simulink model "Simulation"  (R2022b)
settings: Solver=FixedStepAuto  StartTime=0.0  StopTime=param.Tsim  FixedStep=param.tSample  RelTol=1e-3
StopFcn:
  | run animation
  | run plotSol
undefined symbols (not defined in the file or in its folder): f, filterFr, filterFw, filterMr, FR_neg, FR_pos, g1, g2, g3, kFr, ki, kiSeil, kMr, kp, kpSeil, kVSl, kVSx, MR, MRP, param, xi_0
libraries: simulink x10, spsFirstOrderFilterLib x2
(part 3 of 3)

== matlab function Simulation/Flatness-based control1/feedforward control/MATLAB Function ==
  data: z1 input; u1 output; dz1 input; ddz1 input; d3z1 input; z2 input; dz2 input; ddz2 input; d3z2 input; u2 output
function [u1, u2] = feedforward_control(z1, dz1, ddz1, d3z1, z2, dz2, ddz2, d3z2)
%#codegen
% Inputs:
% z1, dz1, ddz1, d3z1: 
% z2, dz2, ddz2, d3z2: 
% Output:
% u1, u2: 


g = 9.81; 


l = z2 / sqrt(1 - (dz1 / dz2)^2); 


dl = (dz2 * sqrt(1 - (dz1 / dz2)^2) - (z2 * dz1 / dz2^2) * (-dz1 * ddz2 + dz2 * ddz1) / sqrt(1 - (dz1 / dz2)^2)) / (1 - (dz1 / dz2)^2);


ddl_num = ...
    ddz2 * sqrt(1 - (dz1 / dz2)^2) ...
    - dz2 * (dz1 / dz2^2) * (-dz1 * ddz2 + dz2 * ddz1) / sqrt(1 - (dz1 / dz2)^2) ...
    - z2 * ((-ddz1 * dz2 + dz1 * ddz2) / dz2^2)^2 ...
    + z2 * (-dz1 / dz2^2) * (-d3z1 * dz2 + 2 * ddz1 * ddz2 - dz1 * d3z2) / sqrt(1 - (dz1 / dz2)^2);
ddl = ddl_num / (1 - (dz1 / dz2)^2);


u1 = d3z1; 


u2 = (1 / l) * ( ...
      -g * (dz1 / dz2) ...  
      - ddz2 * sqrt(1 - (dz1 / dz2)^2) ... 
      - 2 * dz2^2 * dl ...
      - d3z2 * l ... 
      - ddl); 
end

== matlab function Simulation/Flatness-based control1/quasistatic tracking control/Computation of the flat output/MATLAB Function ==
  data: x1 input; z1 output; z2 output; x3 input; x5 input
function [z1, z2] = z(x1, x3, x5)
    % Compute flat outputs
    z1 = x1 + x3 * sin(x5);
    z2 = x3 * cos(x5);
end

== matlab function Simulation/Flatness-based control/trajectory generators/desired trajectory: SP change ==
  data: t input; z1_soll output; T input; z10 input; z20 input; z1T input; z2T input; z2_soll output
function [z1_soll, z2_soll] = fcn(t, T, z10, z20, z1T, z2T)
% Generate smooth trajectory for a single setpoint change
%
% Eingangsvariablen:
% t:    Current simulation time
% T:    Total duration of the trajectory
% z10:  Initial horizontal position
% z20:  Initial vertical position
% z1T:  Target horizontal position
% z2T:  Target vertical position
%
% Ausgangsvariablen:
% z1_soll:  Horizontal trajectory [z1, dz1, ddz1, ...]
% z2_soll:  Vertical trajectory [z2, dz2, ddz2, ...]

% Initialize output variables
z1_soll = zeros(1, 4); % [Position, Velocity, Acceleration, Jerk]
z2_soll = zeros(1, 4);

% Normalize time
tau = t / T; % Scaled time (0 <= tau <= 1)

% Ensure tau is within [0, 1] (handle cases where t > T)
if tau > 1
    tau = 1;
end

% Polynomial coefficients for a fifth-order polynomial
P = [6, -15, 10, 0, 0, 0]; % Standard polynomial for smooth interpolation

% Compute z1 trajectory and its derivatives
z1_soll(1) = z10 + (z1T - z10) * polyval(P, tau); % Position
z1_soll(2) = (z1T - z10) * polyval(polyder(P), tau) / T; % Velocity
z1_soll(3) = (z1T - z10) * polyval(polyder(polyder(P)), tau) / T^2; % Acceleration
z1_soll(4) = (z1T - z10) * polyval(polyder(polyder(polyder(P))), tau) / T^3; % Jerk

% Compute z2 trajectory and its derivatives
z2_soll(1) = z20 + (z2T - z20) * polyval(P, tau); % Position
z2_soll(2) = (z2T - z20) * polyval(polyder(P), tau) / T; % Velocity
z2_soll(3) = (z2T - z20) * polyval(polyder(polyder(P)), tau) / T^2; % Acceleration
z2_soll(4) = (z2T - z20) * polyval(polyder(polyder(polyder(P))), tau) / T^3; % Jerk
end

== matlab function Simulation/Flatness-based control1/quasistatic tracking control/Computation of the flat output/MATLAB Function1 ==
  data: dz1 output; dz2 output; x2 input; x3 input; x4 input; x5 input; x6 input
function [dz1, dz2] = dz(x2, x3, x4, x5, x6)
    dz1 = x2 + x4 * sin(x5) + x3 * x6 * cos(x5);
    dz2 = x4 * cos(x5) - x3 * x6 * sin(x5);
end

== matlab function Simulation/Flatness-based control1/quasistatic tracking control/Computation of the flat output/MATLAB Function2 ==
  data: x3 input; x5 input; x6 input; ddz1 output; ddz2 output; u1 input; u2 input
function [ddz1, ddz2] = ddz(x3, x5, x6, u1, u2)
g=9.81;
    ddz1 = sin(x5) * (u2 + u1 * sin(x5) - x3 * x6^2) - g * sin(x5) * cos(x5);
    ddz2 = cos(x5) * (u2 + u1 * sin(x5) - x3 * x6^2) + g * sin(x5)^2;
end

== matlab function Simulation/System model/Referenzmodell/Unterlagerte v-Regelung/Unterlagerte Regelung Seil/Gravitationskompensation ==
  data: m input; Mg output; g input; rho input
function Mg = fcn(m, g, rho)

Mg = m*g*rho;

== matlab function Simulation/Plot/Lastposition ==
  data: xW input; xL output; l input; phi input; yL output
function [xL, yL] = fcn(xW, l, phi)
    
    xL = xW + sin(phi)*l;
    yL = cos(phi)*l;

end

== matlab function Simulation/Flatness-based control1/quasistatic tracking control/Tracking controller/MATLAB Function ==
  data: ddz1 input; dddz1 input; v1 input; z2 input; u1 output; dz2 input; v2 input; dv2 input; u2 output; ddv2 input
function [u1, u2] = controlInputs(ddz1, dddz1, v1, z2, dz2, v2, dv2, ddv2)
    g = 9.81;
    
    A = (dz2*ddz1 + z2*dddz1)*(v2 - g);
    dA = (v2*ddz1 + dz2*dddz1*2 + z2*v1) * (v2 - g) + (dz2*ddz1 + z2*dddz1) * dv2;
    B = (A - z2*ddz1*dv2) / ((v2 - g)^2);
    dB = ((dA - dz2*ddz1*dv2 - z2*dddz1*dv2 - z2*ddz1*ddv2) * ((v2 - g)^2) ...
        - (A - z2*ddz1*dv2) * 2*(v2 - g)*dv2) ...
        / ((v2 - g)^4);
    x3 = sqrt(z2^2 + (z2*ddz1/(v2 - g))^2);
    dx3 = (2*z2*dz2 + B) / x3;

    u1 = ddz1 - dB;
    u2 = ((2*dz2*dz2 + 2*z2*v2 + dB)*x3...
        - (2*z2*dz2 + B)*dx3)...
        / (x3^2);
end

== matlab function Simulation/Flatness-based control1/quasistatic tracking control/Tracking controller/Tracking controller v1 for xLoad/MATLAB Function ==
  data: z1_star input; dz1_star input; ddz1_star input; dddz1_star input; d4z1_star input; z1 input; v1 output; dz1 input; ddz1 input; dddz1 input; pX01 input; pX02 input; pX03 input; pX04 input
function v1 = newInput_v1(z1_star, dz1_star, ddz1_star, dddz1_star, d4z1_star, z1, dz1, ddz1, dddz1, pX01, pX02, pX03, pX04)
    v1 = d4z1_star - pX01 * (dddz1 - dddz1_star) - pX02 * (ddz1 - ddz1_star) - pX03 * (dz1 - dz1_star) - pX04 * (z1 - z1_star);
end

== matlab function Simulation/Flatness-based control1/quasistatic tracking control/Tracking controller/Tracking controller v2 for yLoad/MATLAB Function ==
  data: z2_star input; dz2_star input; ddz2_star input; dddz2_star input; d4z2_star input; z2 input; v2 output; dz2 input; pY01_QS input; pY02_QS input; dv2 output; ddv2 output
function [v2, dv2, ddv2] = newInput_v2(z2_star, dz2_star, ddz2_star, dddz2_star, d4z2_star, z2, dz2, pY01_QS, pY02_QS)
    v2 = ddz2_star - pY01_QS * (dz2 - dz2_star) - pY02_QS * (z2 - z2_star);
    dv2 = dddz2_star - pY01_QS * (v2 - ddz2_star) - pY02_QS * (dz2 - dz2_star);
    ddv2 = d4z2_star - pY01_QS * (dv2 - dddz2_star) - pY02_QS * (v2 - ddz2_star);
end

== matlab function Simulation/Flatness-based control1/trajectory generators/desired trajectory: Parabola ==
  data: t input; z1_soll output; T input; z10 input; z1T input; a2 input; a1 input; z2_soll output; a0 input
function [z1_soll, z2_soll] = fcn(t, T, z10, z1T, a2, a1, a0)
% Parabola trajectory generator for avoiding obstacles
%
% Eingangsvariablen:
% t:        Current time
% T:        Duration of the trajectory
% z10:      Initial x-coordinate (horizontal position)
% z1T:      Final x-coordinate (horizontal position)
% a2, a1, a0: Coefficients of the parabolic equation z2 = a2*z1^2 + a1*z1 + a0
%
% Ausgangsvariablen:
% z1_soll:  Horizontal trajectory [z1, dz1, ddz1, ...]
% z2_soll:  Vertical trajectory [z2, dz2, ddz2, ...]

% Initialize output variables
z1_soll = zeros(1, 4); % [Position, Velocity, Acceleration, Jerk]
z2_soll = zeros(1, 4);

% Normalize time
tau = t / T; % Scaled time (0 <= tau <= 1)

% Boundary conditions for z1 (horizontal trajectory)
z1_start = z10;
z1_end = z1T;

% Polynomial coefficients for a fifth-order polynomial for z1
P_z1 = [6, -15, 10, 0, 0, 0]; % Scaled polynomial for smooth interpolation

% Compute z1 trajectory and its derivatives
z1_soll(1) = z1_start + (z1_end - z1_start) * polyval(P_z1, tau);
z1_soll(2) = (z1_end - z1_start) * polyval(polyder(P_z1), tau) / T;
z1_soll(3) = (z1_end - z1_start) * polyval(polyder(polyder(P_z1)), tau) / T^2;
z1_soll(4) = (z1_end - z1_start) * polyval(polyder(polyder(polyder(P_z1))), tau) / T^3;

% Compute z2 (vertical trajectory) based on the parabolic equation
z2_soll(1) = a2 * z1_soll(1)^2 + a1 * z1_soll(1) + a0; % Position
z2_soll(2) = 2 * a2 * z1_soll(1) * z1_soll(2) + a1 * z1_soll(2); % Velocity
z2_soll(3) = 2 * a2 * (z1_soll(2)^2 + z1_soll(1) * z1_soll(3)) + a1 * z1_soll(3); % Acceleration
z2_soll(4) = 2 * a2 * (2 * z1_soll(2) * z1_soll(3) + z1_soll(1) * z1_soll(4)) + a1 * z1_soll(4); % Jerk
end

== matlab function Simulation/Flatness-based control1/trajectory generators/desired trajectory: SP change ==
  data: t input; z1_soll output; T input; z10 input; z20 input; z1T input; z2T input; z2_soll output
function [z1_soll, z2_soll] = fcn(t, T, z10, z20, z1T, z2T)
% Generate smooth trajectory for a single setpoint change
%
% Eingangsvariablen:
% t:    Current simulation time
% T:    Total duration of the trajectory
% z10:  Initial horizontal position
% z20:  Initial vertical position
% z1T:  Target horizontal position
% z2T:  Target vertical position
%
% Ausgangsvariablen:
% z1_soll:  Horizontal trajectory [z1, dz1, ddz1, ...]
% z2_soll:  Vertical trajectory [z2, dz2, ddz2, ...]

% Initialize output variables
z1_soll = zeros(1, 4); % [Position, Velocity, Acceleration, Jerk]
z2_soll = zeros(1, 4);

% Normalize time
tau = t / T; % Scaled time (0 <= tau <= 1)

% Ensure tau is within [0, 1] (handle cases where t > T)
if tau > 1
    tau = 1;
end

% Polynomial coefficients for a fifth-order polynomial
P = [6, -15, 10, 0, 0, 0]; % Standard polynomial for smooth interpolation

% Compute z1 trajectory and its derivatives
z1_soll(1) = z10 + (z1T - z10) * polyval(P, tau); 
z1_soll(2) = (z1T - z10) * polyval(polyder(P), tau) / T; 
z1_soll(3) = (z1T - z10) * polyval(polyder(polyder(P)), tau) / T^2; 
z1_soll(4) = (z1T - z10) * polyval(polyder(polyder(polyder(P))), tau) / T^3; 

% Compute z2 trajectory and its derivatives
z2_soll(1) = z20 + (z2T - z20) * polyval(P, tau); 
z2_soll(2) = (z2T - z20) * polyval(polyder(P), tau) / T; 
z2_soll(3) = (z2T - z20) * polyval(polyder(polyder(P)), tau) / T^2; 
z2_soll(4) = (z2T - z20) * polyval(polyder(polyder(polyder(P))), tau) / T^3; 
end

== matlab function Simulation/Flatness-based control1/trajectory generators/desired trajectory: Sequence of SP changes ==
  data: t input; z1_soll output; T input; z10 input; z20 input; z2_soll output; T_task input; x_links input; x_rechts input; y_oben input; y_unten input
function [z1_soll, z2_soll] = fcn(t, T, z10, z20, T_task, x_links, x_rechts, y_oben, y_unten)
% Solltrajektoriengenerator für eine Folge von Arbeitspunktwechseln
%
%%%%%%%%%%%%%%%%%%%%%%%%%%%%%%%%%%%%%%%%%%%%%%%%%%%%%%%%%%%%%%%%%%%%%%%%%%%%%%%%%%%%%%%%%%%%%%
% Eingangsvariablen: 
% t:                    Zeit
% T:                    Zeitdauer eines Arbeitspunktwechsels
% T_task:               Zeitdauer zwischen dem Beginn zweier aufeinanderfolgender Arbeitspunktwechsel
% z10/z20:              Startsollzustand
% x_links, x_rechts:    x-Koordinate der linken/rechten Punkte
% y_oben, y_unten:      y-Koordinate der oberen/unteren Punkte
%
% Ausgangsvariablen:
% z1_soll:  Vektor [z1_soll, dz1_soll, ddz1_soll, ...]
% z2_soll:  Vektor [z2_soll, dz2_soll, ddz2_soll, ...]
%%%%%%%%%%%%%%%%%%%%%%%%%%%%%%%%%%%%%%%%%%%%%%%%%%%%%%%%%%%%%%%%%%%%%%%%%%%%%%%%%%%%%%%%%%%%%%

z1_soll = zeros(1, 4); 
z2_soll = zeros(1, 4);


setpoints = [
    z10, z20;              
    x_links, y_oben;       
    x_links, y_unten;       
    x_rechts, y_oben;       
    x_rechts, y_unten;     
    x_links, y_oben;       
    z10, z20                
];


n_segments = size(setpoints, 1) - 1;
segment_duration = T + T_task;


current_segment = floor(t / segment_duration) + 1;

if current_segment > n_segments
    z1_soll(1) = setpoints(end, 1);
    z2_soll(1) = setpoints(end, 2);
    return;
end

t_local = mod(t, segment_duration);


if t_local > T
    z1_soll(1) = setpoints(current_segment, 1);
    z2_soll(1) = setpoints(current_segment, 2);
    return;
end


z1_start = setpoints(current_segment, 1);
z2_start = setpoints(current_segment, 2);
z1_end = setpoints(current_segment + 1, 1);
z2_end = setpoints(current_segment + 1, 2);

tau = t_local / T;

P = [0, 0, 0, 35, -84, 70, 0, 0, 0, 0];


z1_soll(1) = z1_start + (z1_end - z1_start) * polyval(P, tau);
z1_soll(2) = (z1_end - z1_start) * polyval(polyder(P), tau) / T;
z1_soll(3) = (z1_end - z1_start) * polyval(polyder(polyder(P)), tau) / T^2;
z1_soll(4) = (z1_end - z1_start) * polyval(polyder(polyder(polyder(P))), tau) / T^3;


z2_soll(1) = z2_start + (z2_end - z2_start) * polyval(P, tau);
z2_soll(2) = (z2_end - z2_start) * polyval(polyder(P), tau) / T;
z2_soll(3) = (z2_end - z2_start) * polyval(polyder(polyder(P)), tau) / T^2;
z2_soll(4) = (z2_end - z2_start) * polyval(polyder(polyder(polyder(P))), tau) / T^3;
end

== matlab function Simulation/Flatness-based control/feedforward control/MATLAB Function ==
  data: z1 input; u1 output; dz1 input; ddz1 input; d3z1 input; z2 input; dz2 input; ddz2 input; d3z2 input; u2 output
function [u1, u2] = feedforward_control(z1, dz1, ddz1, d3z1, z2, dz2, ddz2, d3z2)
%#codegen
% Inputs:
% z1, dz1, ddz1, d3z1: 
% z2, dz2, ddz2, d3z2: 
% Output:
% u1, u2: 


g = 9.81; 


l = z2 / sqrt(1 - (dz1 / dz2)^2); 


dl = (dz2 * sqrt(1 - (dz1 / dz2)^2) - (z2 * dz1 / dz2^2) * (-dz1 * ddz2 + dz2 * ddz1) / sqrt(1 - (dz1 / dz2)^2)) / (1 - (dz1 / dz2)^2);


ddl_num = ...
    ddz2 * sqrt(1 - (dz1 / dz2)^2) ...
    - dz2 * (dz1 / dz2^2) * (-dz1 * ddz2 + dz2 * ddz1) / sqrt(1 - (dz1 / dz2)^2) ...
    - z2 * ((-ddz1 * dz2 + dz1 * ddz2) / dz2^2)^2 ...
    + z2 * (-dz1 / dz2^2) * (-d3z1 * dz2 + 2 * ddz1 * ddz2 - dz1 * d3z2) / sqrt(1 - (dz1 / dz2)^2);
ddl = ddl_num / (1 - (dz1 / dz2)^2);


u1 = d3z1; 


u2 = (1 / l) * ( ...
      -g * (dz1 / dz2) ...  
      - ddz2 * sqrt(1 - (dz1 / dz2)^2) ... 
      - 2 * dz2^2 * dl ...
      - d3z2 * l ... 
      - ddl); 
end

== matlab function Simulation/Plot1/Lastposition ==
  data: xW input; xL output; l input; phi input; yL output
function [xL, yL] = fcn(xW, l, phi)
    
    xL = xW + sin(phi)*l;
    yL = cos(phi)*l;

end

== matlab function Simulation/Plot1/yL_Beschraenkung (Parabel) ==
  data: xL input; yL_const output; p0 input; p1 input; p2 input
function yL_const  = fcn(xL, p0, p1, p2)
    % Quadratisches Polynom für die Zustandsbeschränkung p2*x^2+p1*x+p0 (im Horner Schema)
    yL_const = xL * ( p1 + (p2 * xL)) + p0;

end

== matlab function Simulation/System model1/Kinematisches Modell/sys_dgl  ==
  data: x input; u input; dx output
function dx = fcn(x,u)

dx = zeros(length(x), 1);
g = 9.81;

dx(1) = x(2);
dx(2) = u(1);
dx(3) = x(4);
dx(4) = u(2);
dx(5) = x(6);
dx(6) = -((g * sin(x(5)) + cos(x(5))*u(1) + 2 * x(4) * x(6)) / x(3));

== matlab function Simulation/System model1/Referenzmodell/Unterlagerte v-Regelung/Unterlagerte Regelung Seil/Gravitationskompensation ==
  data: m input; Mg output; g input; rho input
function Mg = fcn(m, g, rho)

Mg = m*g*rho;

== matlab function Simulation/System model1/Referenzmodell/Unterlagerte v-Regelung/Unterlagerte Regelung Seil/MATLAB Function7 ==
  data: muT input; c_TT input; c_HT input; omega_0 input; ldt input; Rho input; Mr output
function Mr = fcn(muT, c_TT, c_HT, omega_0, ldt, Rho)


Mr = -(muT*(-ldt/Rho)+c_TT*sign(-ldt/Rho)+(c_HT-c_TT)*sign(-ldt/Rho)*exp((-ldt^2*omega_0^2)/Rho^2));

% Mr = -(muT*(-ldt/Rho));

== matlab function Simulation/System model1/Referenzmodell/Unterlagerte v-Regelung/Unterlagerte Regelung Wagen/MATLAB Function2 ==
  data: mu_W_pos input; c_TW_pos input; c_HW_pos input; v_0_pos input; xdt input; Fr output
function Fr = fcn(mu_W_pos, c_TW_pos, c_HW_pos, v_0_pos, xdt)

%     Fr = -(mu_W_pos*xdt +(c_HW_pos-c_TW_pos)*sign(xdt)*exp(-xdt^2/v_0_pos^2) + c_TW_pos*sign(xdt));
    
    Fr = -(mu_W_pos*xdt + c_TW_pos*sign(xdt));

== matlab function Simulation/Flatness-based control/quasistatic tracking control/Computation of the flat output/MATLAB Function ==
  data: x1 input; z1 output; z2 output; x3 input; x5 input
function [z1, z2] = z(x1, x3, x5)
    % Compute flat outputs
    z1 = x1 + x3 * sin(x5);
    z2 = x3 * cos(x5);
end

== matlab function Simulation/Flatness-based control/quasistatic tracking control/Computation of the flat output/MATLAB Function1 ==
  data: dz1 output; dz2 output; x2 input; x3 input; x4 input; x5 input; x6 input
function [dz1, dz2] = dz(x2, x3, x4, x5, x6)
    dz1 = x2 + x4 * sin(x5) + x3 * x6 * cos(x5);
    dz2 = x4 * cos(x5) - x3 * x6 * sin(x5);
end

== matlab function Simulation/Flatness-based control/trajectory generators/desired trajectory: Sequence of SP changes ==
  data: t input; z1_soll output; T input; z10 input; z20 input; z2_soll output; T_task input; x_links input; x_rechts input; y_oben input; y_unten input
function [z1_soll, z2_soll] = fcn(t, T, z10, z20, T_task, x_links, x_rechts, y_oben, y_unten)
% Solltrajektoriengenerator für eine Folge von Arbeitspunktwechseln
%
%%%%%%%%%%%%%%%%%%%%%%%%%%%%%%%%%%%%%%%%%%%%%%%%%%%%%%%%%%%%%%%%%%%%%%%%%%%%%%%%%%%%%%%%%%%%%%
% Eingangsvariablen: 
% t:                    Zeit
% T:                    Zeitdauer eines Arbeitspunktwechsels
% T_task:               Zeitdauer zwischen dem Beginn zweier aufeinanderfolgender Arbeitspunktwechsel
% z10/z20:              Startsollzustand
% x_links, x_rechts:    x-Koordinate der linken/rechten Punkte
% y_oben, y_unten:      y-Koordinate der oberen/unteren Punkte
%
% Ausgangsvariablen:
% z1_soll:  Vektor [z1_soll, dz1_soll, ddz1_soll, ...]
% z2_soll:  Vektor [z2_soll, dz2_soll, ddz2_soll, ...]
%%%%%%%%%%%%%%%%%%%%%%%%%%%%%%%%%%%%%%%%%%%%%%%%%%%%%%%%%%%%%%%%%%%%%%%%%%%%%%%%%%%%%%%%%%%%%%

z1_soll = zeros(1, 4); 
z2_soll = zeros(1, 4);


setpoints = [
    z10, z20;              
    x_links, y_oben;       
    x_links, y_unten;       
    x_rechts, y_oben;       
    x_rechts, y_unten;     
    x_links, y_oben;       
    z10, z20                
];


n_segments = size(setpoints, 1) - 1;
segment_duration = T + T_task;


current_segment = floor(t / segment_duration) + 1;

if current_segment > n_segments
    z1_soll(1) = setpoints(end, 1);
    z2_soll(1) = setpoints(end, 2);
    return;
end

t_local = mod(t, segment_duration);


if t_local > T
    z1_soll(1) = setpoints(current_segment, 1);
    z2_soll(1) = setpoints(current_segment, 2);
    return;
end


z1_start = setpoints(current_segment, 1);
z2_start = setpoints(current_segment, 2);
z1_end = setpoints(current_segment + 1, 1);
z2_end = setpoints(current_segment + 1, 2);

tau = t_local / T;

P = [0, 0, 0, 35, -84, 70, 0, 0, 0, 0];


z1_soll(1) = z1_start + (z1_end - z1_start) * polyval(P, tau);
z1_soll(2) = (z1_end - z1_start) * polyval(polyder(P), tau) / T;
z1_soll(3) = (z1_end - z1_start) * polyval(polyder(polyder(P)), tau) / T^2;
z1_soll(4) = (z1_end - z1_start) * polyval(polyder(polyder(polyder(P))), tau) / T^3;


z2_soll(1) = z2_start + (z2_end - z2_start) * polyval(P, tau);
z2_soll(2) = (z2_end - z2_start) * polyval(polyder(P), tau) / T;
z2_soll(3) = (z2_end - z2_start) * polyval(polyder(polyder(P)), tau) / T^2;
z2_soll(4) = (z2_end - z2_start) * polyval(polyder(polyder(polyder(P))), tau) / T^3;
end
